simulink model "sm_car"  (R2025b)
settings: Solver=ode23t  StartTime=0.0  StopTime=100  MaxStep=0.4  RelTol=1e-3  AbsTol=1e-3  EnableMultiTasking=on
PreLoadFcn:
  | % Due to usability issue in Repeating Sequence block
  | warning('off','Simulink:Masking:Invalid');
  | 
  | % Eliminate unnecessary warnings in inactive variants
  | % Warnings generated only if you click through inactive variant
  | warning('off','MATLAB:nonExistentField');
  | warning('off','Simulink:Parameters:BlkParamUndefined');
PostLoadFcn:
  | set_param([bdroot '/Vehicle'],'popup_trailer','Off')
  | warning('off','sm:sli:setup:compile:LocalSolverNotSupported')
  | %sm_car_config_maneuver(bdroot,'WOT Braking');
  | sm_car_config_vehicle(bdroot,'false');
  | sm_car_config_logging(bdroot);
InitFcn:
  | sm_car_config_camera;
  | Vehicle = sm_car_vehcfg_checkConfig(Vehicle);
  | sm_car_check_tire_model(bdroot);
StartFcn:
  | tic;
StopFcn:
  | Elapsed_Sim_Time = toc;
  | % disp(['Elapsed Sim Time = ' num2str(Elapsed_Sim_Time)]);
undefined symbols (not defined in the file): Axle1D, AxleIn, Camera, Control, Driver, Init, Maneuver, Pedal, Scene, ShaftL1, ShaftL2, ShaftR1, ShaftR2, Visual, X, xy_data_car_side, Y, Z
libraries: sm_lib x255, fl_lib x191, nesl_utility x149, simulink x23, sdl_lib x14, simulink_extras x8, SimscapeFluids_lib x7, Scene_Utilities x6, Tire_1x2x x4, ee_lib x3, Linkage x2, fuzblock x1
(part 3 of 19)

== system sm_car/Camera Frames/Transform FixO RR ==
  Transform Camera Frame : sm_lib/Frames and Transforms/Rigid Transform  RotationMethod=RotationSequence  FollAlignAxisA=+X  BaseAlignAxisA=+Y  FollAlignAxisB=+Y  BaseAlignAxisB=+Z  RotationStandardAxis=+Z  RotationAngle=0.0  RotationAngleUnits=deg  RotationArbitraryAxis=[0 0 1]  RotationSequenceAxes=FollowerAxes  RotationSequence=ZYX  RotationSequenceAngles=CF.a.Value(3:-1:1)  RotationSequenceAnglesUnits=deg  RotationMatrix=[1 0 0; 0 1 0; 0 0 1]  Quaternion=[1 0 0 0]  TranslationMethod=Cartesian  TranslationCartesianOffset=CF.s.Value  TranslationCartesianOffsetUnits=m  TranslationStandardAxis=+Z  TranslationStandardOffset=0  TranslationStandardOffsetUnits=m  TranslationROffset=0  TranslationROffsetUnits=m  TranslationThetaOffset=0  TranslationThetaOffsetUnits=deg  TranslationZOffset=0  TranslationZOffsetUnits=m
  B : PMIOPort  Side=Left
  F : PMIOPort  Port=2  Side=Right
  connections:
  Transform Camera Frame/RConn1 -- F/RConn1
  Transform Camera Frame/LConn1 -- B/RConn1

== system sm_car/Camera Frames/Transform FixO Rear ==
  Transform Camera Frame : sm_lib/Frames and Transforms/Rigid Transform  RotationMethod=RotationSequence  FollAlignAxisA=+X  BaseAlignAxisA=+Y  FollAlignAxisB=+Y  BaseAlignAxisB=+Z  RotationStandardAxis=+Z  RotationAngle=0.0  RotationAngleUnits=deg  RotationArbitraryAxis=[0 0 1]  RotationSequenceAxes=FollowerAxes  RotationSequence=ZYX  RotationSequenceAngles=CF.a.Value(3:-1:1)  RotationSequenceAnglesUnits=deg  RotationMatrix=[1 0 0; 0 1 0; 0 0 1]  Quaternion=[1 0 0 0]  TranslationMethod=Cartesian  TranslationCartesianOffset=CF.s.Value  TranslationCartesianOffsetUnits=m  TranslationStandardAxis=+Z  TranslationStandardOffset=0  TranslationStandardOffsetUnits=m  TranslationROffset=0  TranslationROffsetUnits=m  TranslationThetaOffset=0  TranslationThetaOffsetUnits=deg  TranslationZOffset=0  TranslationZOffsetUnits=m
  B : PMIOPort  Side=Left
  F : PMIOPort  Port=2  Side=Right
  connections:
  Transform Camera Frame/RConn1 -- F/RConn1
  Transform Camera Frame/LConn1 -- B/RConn1

== system sm_car/Camera Frames/Transform FixO Right ==
  Transform Camera Frame : sm_lib/Frames and Transforms/Rigid Transform  RotationMethod=RotationSequence  FollAlignAxisA=+X  BaseAlignAxisA=+Y  FollAlignAxisB=+Y  BaseAlignAxisB=+Z  RotationStandardAxis=+Z  RotationAngle=0.0  RotationAngleUnits=deg  RotationArbitraryAxis=[0 0 1]  RotationSequenceAxes=FollowerAxes  RotationSequence=ZYX  RotationSequenceAngles=CF.a.Value(3:-1:1)  RotationSequenceAnglesUnits=deg  RotationMatrix=[1 0 0; 0 1 0; 0 0 1]  Quaternion=[1 0 0 0]  TranslationMethod=Cartesian  TranslationCartesianOffset=CF.s.Value  TranslationCartesianOffsetUnits=m  TranslationStandardAxis=+Z  TranslationStandardOffset=0  TranslationStandardOffsetUnits=m  TranslationROffset=0  TranslationROffsetUnits=m  TranslationThetaOffset=0  TranslationThetaOffsetUnits=deg  TranslationZOffset=0  TranslationZOffsetUnits=m
  B : PMIOPort  Side=Left
  F : PMIOPort  Port=2  Side=Right
  connections:
  Transform Camera Frame/RConn1 -- F/RConn1
  Transform Camera Frame/LConn1 -- B/RConn1

== system sm_car/Camera Frames/Transform FixO Top ==
  Transform Camera Frame : sm_lib/Frames and Transforms/Rigid Transform  RotationMethod=RotationSequence  FollAlignAxisA=+X  BaseAlignAxisA=+Y  FollAlignAxisB=+Y  BaseAlignAxisB=+Z  RotationStandardAxis=+Z  RotationAngle=0.0  RotationAngleUnits=deg  RotationArbitraryAxis=[0 0 1]  RotationSequenceAxes=FollowerAxes  RotationSequence=ZYX  RotationSequenceAngles=CF.a.Value(3:-1:1)  RotationSequenceAnglesUnits=deg  RotationMatrix=[1 0 0; 0 1 0; 0 0 1]  Quaternion=[1 0 0 0]  TranslationMethod=Cartesian  TranslationCartesianOffset=CF.s.Value  TranslationCartesianOffsetUnits=m  TranslationStandardAxis=+Z  TranslationStandardOffset=0  TranslationStandardOffsetUnits=m  TranslationROffset=0  TranslationROffsetUnits=m  TranslationThetaOffset=0  TranslationThetaOffsetUnits=deg  TranslationZOffset=0  TranslationZOffsetUnits=m
  B : PMIOPort  Side=Left
  F : PMIOPort  Port=2  Side=Right
  connections:
  Transform Camera Frame/RConn1 -- F/RConn1
  Transform Camera Frame/LConn1 -- B/RConn1

== system sm_car/Camera Frames/Transform Front ==
  Transform Camera Frame : sm_lib/Frames and Transforms/Rigid Transform  RotationMethod=RotationSequence  FollAlignAxisA=+X  BaseAlignAxisA=+Y  FollAlignAxisB=+Y  BaseAlignAxisB=+Z  RotationStandardAxis=+Z  RotationAngle=0.0  RotationAngleUnits=deg  RotationArbitraryAxis=[0 0 1]  RotationSequenceAxes=FollowerAxes  RotationSequence=ZYX  RotationSequenceAngles=CF.a.Value(3:-1:1)  RotationSequenceAnglesUnits=deg  RotationMatrix=[1 0 0; 0 1 0; 0 0 1]  Quaternion=[1 0 0 0]  TranslationMethod=Cartesian  TranslationCartesianOffset=CF.s.Value  TranslationCartesianOffsetUnits=m  TranslationStandardAxis=+Z  TranslationStandardOffset=0  TranslationStandardOffsetUnits=m  TranslationROffset=0  TranslationROffsetUnits=m  TranslationThetaOffset=0  TranslationThetaOffsetUnits=deg  TranslationZOffset=0  TranslationZOffsetUnits=m
  B : PMIOPort  Side=Left
  F : PMIOPort  Port=2  Side=Right
  connections:
  Transform Camera Frame/RConn1 -- F/RConn1
  Transform Camera Frame/LConn1 -- B/RConn1

== system sm_car/Camera Frames/Transform Left ==
  Transform Camera Frame : sm_lib/Frames and Transforms/Rigid Transform  RotationMethod=RotationSequence  FollAlignAxisA=+X  BaseAlignAxisA=+Y  FollAlignAxisB=+Y  BaseAlignAxisB=+Z  RotationStandardAxis=+Z  RotationAngle=0.0  RotationAngleUnits=deg  RotationArbitraryAxis=[0 0 1]  RotationSequenceAxes=FollowerAxes  RotationSequence=ZYX  RotationSequenceAngles=CF.a.Value(3:-1:1)  RotationSequenceAnglesUnits=deg  RotationMatrix=[1 0 0; 0 1 0; 0 0 1]  Quaternion=[1 0 0 0]  TranslationMethod=Cartesian  TranslationCartesianOffset=CF.s.Value  TranslationCartesianOffsetUnits=m  TranslationStandardAxis=+Z  TranslationStandardOffset=0  TranslationStandardOffsetUnits=m  TranslationROffset=0  TranslationROffsetUnits=m  TranslationThetaOffset=0  TranslationThetaOffsetUnits=deg  TranslationZOffset=0  TranslationZOffsetUnits=m
  B : PMIOPort  Side=Left
  F : PMIOPort  Port=2  Side=Right
  connections:
  Transform Camera Frame/RConn1 -- F/RConn1
  Transform Camera Frame/LConn1 -- B/RConn1

== system sm_car/Camera Frames/Transform RL ==
  Transform Camera Frame : sm_lib/Frames and Transforms/Rigid Transform  RotationMethod=RotationSequence  FollAlignAxisA=+X  BaseAlignAxisA=+Y  FollAlignAxisB=+Y  BaseAlignAxisB=+Z  RotationStandardAxis=+Z  RotationAngle=0.0  RotationAngleUnits=deg  RotationArbitraryAxis=[0 0 1]  RotationSequenceAxes=FollowerAxes  RotationSequence=ZYX  RotationSequenceAngles=CF.a.Value(3:-1:1)  RotationSequenceAnglesUnits=deg  RotationMatrix=[1 0 0; 0 1 0; 0 0 1]  Quaternion=[1 0 0 0]  TranslationMethod=Cartesian  TranslationCartesianOffset=CF.s.Value  TranslationCartesianOffsetUnits=m  TranslationStandardAxis=+Z  TranslationStandardOffset=0  TranslationStandardOffsetUnits=m  TranslationROffset=0  TranslationROffsetUnits=m  TranslationThetaOffset=0  TranslationThetaOffsetUnits=deg  TranslationZOffset=0  TranslationZOffsetUnits=m
  B : PMIOPort  Side=Left
  F : PMIOPort  Port=2  Side=Right
  connections:
  Transform Camera Frame/RConn1 -- F/RConn1
  Transform Camera Frame/LConn1 -- B/RConn1

== system sm_car/Camera Frames/Transform RR ==
  Transform Camera Frame : sm_lib/Frames and Transforms/Rigid Transform  RotationMethod=RotationSequence  FollAlignAxisA=+X  BaseAlignAxisA=+Y  FollAlignAxisB=+Y  BaseAlignAxisB=+Z  RotationStandardAxis=+Z  RotationAngle=0.0  RotationAngleUnits=deg  RotationArbitraryAxis=[0 0 1]  RotationSequenceAxes=FollowerAxes  RotationSequence=ZYX  RotationSequenceAngles=CF.a.Value(3:-1:1)  RotationSequenceAnglesUnits=deg  RotationMatrix=[1 0 0; 0 1 0; 0 0 1]  Quaternion=[1 0 0 0]  TranslationMethod=Cartesian  TranslationCartesianOffset=CF.s.Value  TranslationCartesianOffsetUnits=m  TranslationStandardAxis=+Z  TranslationStandardOffset=0  TranslationStandardOffsetUnits=m  TranslationROffset=0  TranslationROffsetUnits=m  TranslationThetaOffset=0  TranslationThetaOffsetUnits=deg  TranslationZOffset=0  TranslationZOffsetUnits=m
  B : PMIOPort  Side=Left
  F : PMIOPort  Port=2  Side=Right
  connections:
  Transform Camera Frame/RConn1 -- F/RConn1
  Transform Camera Frame/LConn1 -- B/RConn1

== system sm_car/Camera Frames/Transform Rear ==
  Transform Camera Frame : sm_lib/Frames and Transforms/Rigid Transform  RotationMethod=RotationSequence  FollAlignAxisA=+X  BaseAlignAxisA=+Y  FollAlignAxisB=+Y  BaseAlignAxisB=+Z  RotationStandardAxis=+Z  RotationAngle=0.0  RotationAngleUnits=deg  RotationArbitraryAxis=[0 0 1]  RotationSequenceAxes=FollowerAxes  RotationSequence=ZYX  RotationSequenceAngles=CF.a.Value(3:-1:1)  RotationSequenceAnglesUnits=deg  RotationMatrix=[1 0 0; 0 1 0; 0 0 1]  Quaternion=[1 0 0 0]  TranslationMethod=Cartesian  TranslationCartesianOffset=CF.s.Value  TranslationCartesianOffsetUnits=m  TranslationStandardAxis=+Z  TranslationStandardOffset=0  TranslationStandardOffsetUnits=m  TranslationROffset=0  TranslationROffsetUnits=m  TranslationThetaOffset=0  TranslationThetaOffsetUnits=deg  TranslationZOffset=0  TranslationZOffsetUnits=m
  B : PMIOPort  Side=Left
  F : PMIOPort  Port=2  Side=Right
  connections:
  Transform Camera Frame/RConn1 -- F/RConn1
  Transform Camera Frame/LConn1 -- B/RConn1

== system sm_car/Camera Frames/Transform Right ==
  Transform Camera Frame : sm_lib/Frames and Transforms/Rigid Transform  RotationMethod=RotationSequence  FollAlignAxisA=+X  BaseAlignAxisA=+Y  FollAlignAxisB=+Y  BaseAlignAxisB=+Z  RotationStandardAxis=+Z  RotationAngle=0.0  RotationAngleUnits=deg  RotationArbitraryAxis=[0 0 1]  RotationSequenceAxes=FollowerAxes  RotationSequence=ZYX  RotationSequenceAngles=CF.a.Value(3:-1:1)  RotationSequenceAnglesUnits=deg  RotationMatrix=[1 0 0; 0 1 0; 0 0 1]  Quaternion=[1 0 0 0]  TranslationMethod=Cartesian  TranslationCartesianOffset=CF.s.Value  TranslationCartesianOffsetUnits=m  TranslationStandardAxis=+Z  TranslationStandardOffset=0  TranslationStandardOffsetUnits=m  TranslationROffset=0  TranslationROffsetUnits=m  TranslationThetaOffset=0  TranslationThetaOffsetUnits=deg  TranslationZOffset=0  TranslationZOffsetUnits=m
  B : PMIOPort  Side=Left
  F : PMIOPort  Port=2  Side=Right
  connections:
  Transform Camera Frame/RConn1 -- F/RConn1
  Transform Camera Frame/LConn1 -- B/RConn1

== system sm_car/Camera Frames/Transform SuspF ==
  Transform Camera Frame : sm_lib/Frames and Transforms/Rigid Transform  RotationMethod=RotationSequence  FollAlignAxisA=+X  BaseAlignAxisA=+Y  FollAlignAxisB=+Y  BaseAlignAxisB=+Z  RotationStandardAxis=+Z  RotationAngle=0.0  RotationAngleUnits=deg  RotationArbitraryAxis=[0 0 1]  RotationSequenceAxes=FollowerAxes  RotationSequence=ZYX  RotationSequenceAngles=CF.a.Value(3:-1:1)  RotationSequenceAnglesUnits=deg  RotationMatrix=[1 0 0; 0 1 0; 0 0 1]  Quaternion=[1 0 0 0]  TranslationMethod=Cartesian  TranslationCartesianOffset=CF.s.Value  TranslationCartesianOffsetUnits=m  TranslationStandardAxis=+Z  TranslationStandardOffset=0  TranslationStandardOffsetUnits=m  TranslationROffset=0  TranslationROffsetUnits=m  TranslationThetaOffset=0  TranslationThetaOffsetUnits=deg  TranslationZOffset=0  TranslationZOffsetUnits=m
  B : PMIOPort  Side=Left
  F : PMIOPort  Port=2  Side=Right
  connections:
  Transform Camera Frame/RConn1 -- F/RConn1
  Transform Camera Frame/LConn1 -- B/RConn1

== system sm_car/Camera Frames/Transform SuspR ==
  Transform Camera Frame : sm_lib/Frames and Transforms/Rigid Transform  RotationMethod=RotationSequence  FollAlignAxisA=+X  BaseAlignAxisA=+Y  FollAlignAxisB=+Y  BaseAlignAxisB=+Z  RotationStandardAxis=+Z  RotationAngle=0.0  RotationAngleUnits=deg  RotationArbitraryAxis=[0 0 1]  RotationSequenceAxes=FollowerAxes  RotationSequence=ZYX  RotationSequenceAngles=CF.a.Value(3:-1:1)  RotationSequenceAnglesUnits=deg  RotationMatrix=[1 0 0; 0 1 0; 0 0 1]  Quaternion=[1 0 0 0]  TranslationMethod=Cartesian  TranslationCartesianOffset=CF.s.Value  TranslationCartesianOffsetUnits=m  TranslationStandardAxis=+Z  TranslationStandardOffset=0  TranslationStandardOffsetUnits=m  TranslationROffset=0  TranslationROffsetUnits=m  TranslationThetaOffset=0  TranslationThetaOffsetUnits=deg  TranslationZOffset=0  TranslationZOffsetUnits=m
  B : PMIOPort  Side=Left
  F : PMIOPort  Port=2  Side=Right
  connections:
  Transform Camera Frame/RConn1 -- F/RConn1
  Transform Camera Frame/LConn1 -- B/RConn1

== system sm_car/Camera Frames/Transform Top ==
  Transform Camera Frame : sm_lib/Frames and Transforms/Rigid Transform  RotationMethod=RotationSequence  FollAlignAxisA=+X  BaseAlignAxisA=+Y  FollAlignAxisB=+Y  BaseAlignAxisB=+Z  RotationStandardAxis=+Z  RotationAngle=0.0  RotationAngleUnits=deg  RotationArbitraryAxis=[0 0 1]  RotationSequenceAxes=FollowerAxes  RotationSequence=ZYX  RotationSequenceAngles=CF.a.Value(3:-1:1)  RotationSequenceAnglesUnits=deg  RotationMatrix=[1 0 0; 0 1 0; 0 0 1]  Quaternion=[1 0 0 0]  TranslationMethod=Cartesian  TranslationCartesianOffset=CF.s.Value  TranslationCartesianOffsetUnits=m  TranslationStandardAxis=+Z  TranslationStandardOffset=0  TranslationStandardOffsetUnits=m  TranslationROffset=0  TranslationROffsetUnits=m  TranslationThetaOffset=0  TranslationThetaOffsetUnits=deg  TranslationZOffset=0  TranslationZOffsetUnits=m
  B : PMIOPort  Side=Left
  F : PMIOPort  Port=2  Side=Right
  connections:
  Transform Camera Frame/RConn1 -- F/RConn1
  Transform Camera Frame/LConn1 -- B/RConn1

== system sm_car/Camera Frames/Transform View Seat FL ==
  Transform Camera Frame : sm_lib/Frames and Transforms/Rigid Transform  RotationMethod=RotationSequence  FollAlignAxisA=+X  BaseAlignAxisA=+Y  FollAlignAxisB=+Y  BaseAlignAxisB=+Z  RotationStandardAxis=+Z  RotationAngle=0.0  RotationAngleUnits=deg  RotationArbitraryAxis=[0 0 1]  RotationSequenceAxes=FollowerAxes  RotationSequence=ZYX  RotationSequenceAngles=CF.a.Value(3:-1:1)  RotationSequenceAnglesUnits=deg  RotationMatrix=[1 0 0; 0 1 0; 0 0 1]  Quaternion=[1 0 0 0]  TranslationMethod=Cartesian  TranslationCartesianOffset=CF.s.Value  TranslationCartesianOffsetUnits=m  TranslationStandardAxis=+Z  TranslationStandardOffset=0  TranslationStandardOffsetUnits=m  TranslationROffset=0  TranslationROffsetUnits=m  TranslationThetaOffset=0  TranslationThetaOffsetUnits=deg  TranslationZOffset=0  TranslationZOffsetUnits=m
  B : PMIOPort  Side=Left
  F : PMIOPort  Port=2  Side=Right
  connections:
  Transform Camera Frame/RConn1 -- F/RConn1
  Transform Camera Frame/LConn1 -- B/RConn1

== system sm_car/Camera Frames/Transform View Seat FR ==
  Transform Camera Frame : sm_lib/Frames and Transforms/Rigid Transform  RotationMethod=RotationSequence  FollAlignAxisA=+X  BaseAlignAxisA=+Y  FollAlignAxisB=+Y  BaseAlignAxisB=+Z  RotationStandardAxis=+Z  RotationAngle=0.0  RotationAngleUnits=deg  RotationArbitraryAxis=[0 0 1]  RotationSequenceAxes=FollowerAxes  RotationSequence=ZYX  RotationSequenceAngles=CF.a.Value(3:-1:1)  RotationSequenceAnglesUnits=deg  RotationMatrix=[1 0 0; 0 1 0; 0 0 1]  Quaternion=[1 0 0 0]  TranslationMethod=Cartesian  TranslationCartesianOffset=CF.s.Value  TranslationCartesianOffsetUnits=m  TranslationStandardAxis=+Z  TranslationStandardOffset=0  TranslationStandardOffsetUnits=m  TranslationROffset=0  TranslationROffsetUnits=m  TranslationThetaOffset=0  TranslationThetaOffsetUnits=deg  TranslationZOffset=0  TranslationZOffsetUnits=m
  B : PMIOPort  Side=Left
  F : PMIOPort  Port=2  Side=Right
  connections:
  Transform Camera Frame/RConn1 -- F/RConn1
  Transform Camera Frame/LConn1 -- B/RConn1

== system sm_car/Camera Frames/Transform View Susp FL ==
  Transform Camera Frame : sm_lib/Frames and Transforms/Rigid Transform  RotationMethod=RotationSequence  FollAlignAxisA=+X  BaseAlignAxisA=+Y  FollAlignAxisB=+Y  BaseAlignAxisB=+Z  RotationStandardAxis=+Z  RotationAngle=0.0  RotationAngleUnits=deg  RotationArbitraryAxis=[0 0 1]  RotationSequenceAxes=FollowerAxes  RotationSequence=ZYX  RotationSequenceAngles=CF.a.Value(3:-1:1)  RotationSequenceAnglesUnits=deg  RotationMatrix=[1 0 0; 0 1 0; 0 0 1]  Quaternion=[1 0 0 0]  TranslationMethod=Cartesian  TranslationCartesianOffset=CF.s.Value  TranslationCartesianOffsetUnits=m  TranslationStandardAxis=+Z  TranslationStandardOffset=0  TranslationStandardOffsetUnits=m  TranslationROffset=0  TranslationROffsetUnits=m  TranslationThetaOffset=0  TranslationThetaOffsetUnits=deg  TranslationZOffset=0  TranslationZOffsetUnits=m
  B : PMIOPort  Side=Left
  F : PMIOPort  Port=2  Side=Right
  connections:
  Transform Camera Frame/RConn1 -- F/RConn1
  Transform Camera Frame/LConn1 -- B/RConn1

== system sm_car/Camera Frames/Transform View Susp FR ==
  Transform Camera Frame : sm_lib/Frames and Transforms/Rigid Transform  RotationMethod=RotationSequence  FollAlignAxisA=+X  BaseAlignAxisA=+Y  FollAlignAxisB=+Y  BaseAlignAxisB=+Z  RotationStandardAxis=+Z  RotationAngle=0.0  RotationAngleUnits=deg  RotationArbitraryAxis=[0 0 1]  RotationSequenceAxes=FollowerAxes  RotationSequence=ZYX  RotationSequenceAngles=CF.a.Value(3:-1:1)  RotationSequenceAnglesUnits=deg  RotationMatrix=[1 0 0; 0 1 0; 0 0 1]  Quaternion=[1 0 0 0]  TranslationMethod=Cartesian  TranslationCartesianOffset=CF.s.Value  TranslationCartesianOffsetUnits=m  TranslationStandardAxis=+Z  TranslationStandardOffset=0  TranslationStandardOffsetUnits=m  TranslationROffset=0  TranslationROffsetUnits=m  TranslationThetaOffset=0  TranslationThetaOffsetUnits=deg  TranslationZOffset=0  TranslationZOffsetUnits=m
  B : PMIOPort  Side=Left
  F : PMIOPort  Port=2  Side=Right
  connections:
  Transform Camera Frame/RConn1 -- F/RConn1
  Transform Camera Frame/LConn1 -- B/RConn1

== system sm_car/Camera Frames/Transform View Susp RL ==
  Transform Camera Frame : sm_lib/Frames and Transforms/Rigid Transform  RotationMethod=RotationSequence  FollAlignAxisA=+X  BaseAlignAxisA=+Y  FollAlignAxisB=+Y  BaseAlignAxisB=+Z  RotationStandardAxis=+Z  RotationAngle=0.0  RotationAngleUnits=deg  RotationArbitraryAxis=[0 0 1]  RotationSequenceAxes=FollowerAxes  RotationSequence=ZYX  RotationSequenceAngles=CF.a.Value(3:-1:1)  RotationSequenceAnglesUnits=deg  RotationMatrix=[1 0 0; 0 1 0; 0 0 1]  Quaternion=[1 0 0 0]  TranslationMethod=Cartesian  TranslationCartesianOffset=CF.s.Value  TranslationCartesianOffsetUnits=m  TranslationStandardAxis=+Z  TranslationStandardOffset=0  TranslationStandardOffsetUnits=m  TranslationROffset=0  TranslationROffsetUnits=m  TranslationThetaOffset=0  TranslationThetaOffsetUnits=deg  TranslationZOffset=0  TranslationZOffsetUnits=m
  B : PMIOPort  Side=Left
  F : PMIOPort  Port=2  Side=Right
  connections:
  Transform Camera Frame/RConn1 -- F/RConn1
  Transform Camera Frame/LConn1 -- B/RConn1

== system sm_car/Camera Frames/Transform View Susp RR ==
  Transform Camera Frame : sm_lib/Frames and Transforms/Rigid Transform  RotationMethod=RotationSequence  FollAlignAxisA=+X  BaseAlignAxisA=+Y  FollAlignAxisB=+Y  BaseAlignAxisB=+Z  RotationStandardAxis=+Z  RotationAngle=0.0  RotationAngleUnits=deg  RotationArbitraryAxis=[0 0 1]  RotationSequenceAxes=FollowerAxes  RotationSequence=ZYX  RotationSequenceAngles=CF.a.Value(3:-1:1)  RotationSequenceAnglesUnits=deg  RotationMatrix=[1 0 0; 0 1 0; 0 0 1]  Quaternion=[1 0 0 0]  TranslationMethod=Cartesian  TranslationCartesianOffset=CF.s.Value  TranslationCartesianOffsetUnits=m  TranslationStandardAxis=+Z  TranslationStandardOffset=0  TranslationStandardOffsetUnits=m  TranslationROffset=0  TranslationROffsetUnits=m  TranslationThetaOffset=0  TranslationThetaOffsetUnits=deg  TranslationZOffset=0  TranslationZOffsetUnits=m
  B : PMIOPort  Side=Left
  F : PMIOPort  Port=2  Side=Right
  connections:
  Transform Camera Frame/RConn1 -- F/RConn1
  Transform Camera Frame/LConn1 -- B/RConn1

== system sm_car/Camera Frames/Transform Wheel FL ==
  Transform Camera Frame : sm_lib/Frames and Transforms/Rigid Transform  RotationMethod=RotationSequence  FollAlignAxisA=+X  BaseAlignAxisA=+Y  FollAlignAxisB=+Y  BaseAlignAxisB=+Z  RotationStandardAxis=+Z  RotationAngle=0.0  RotationAngleUnits=deg  RotationArbitraryAxis=[0 0 1]  RotationSequenceAxes=FollowerAxes  RotationSequence=ZYX  RotationSequenceAngles=CF.a.Value(3:-1:1)  RotationSequenceAnglesUnits=deg  RotationMatrix=[1 0 0; 0 1 0; 0 0 1]  Quaternion=[1 0 0 0]  TranslationMethod=Cartesian  TranslationCartesianOffset=CF.s.Value  TranslationCartesianOffsetUnits=m  TranslationStandardAxis=+Z  TranslationStandardOffset=0  TranslationStandardOffsetUnits=m  TranslationROffset=0  TranslationROffsetUnits=m  TranslationThetaOffset=0  TranslationThetaOffsetUnits=deg  TranslationZOffset=0  TranslationZOffsetUnits=m
  B : PMIOPort  Side=Left
  F : PMIOPort  Port=2  Side=Right
  connections:
  Transform Camera Frame/RConn1 -- F/RConn1
  Transform Camera Frame/LConn1 -- B/RConn1

== system sm_car/Camera Frames/Transform Wheel FR ==
  Transform Camera Frame : sm_lib/Frames and Transforms/Rigid Transform  RotationMethod=RotationSequence  FollAlignAxisA=+X  BaseAlignAxisA=+Y  FollAlignAxisB=+Y  BaseAlignAxisB=+Z  RotationStandardAxis=+Z  RotationAngle=0.0  RotationAngleUnits=deg  RotationArbitraryAxis=[0 0 1]  RotationSequenceAxes=FollowerAxes  RotationSequence=ZYX  RotationSequenceAngles=CF.a.Value(3:-1:1)  RotationSequenceAnglesUnits=deg  RotationMatrix=[1 0 0; 0 1 0; 0 0 1]  Quaternion=[1 0 0 0]  TranslationMethod=Cartesian  TranslationCartesianOffset=CF.s.Value  TranslationCartesianOffsetUnits=m  TranslationStandardAxis=+Z  TranslationStandardOffset=0  TranslationStandardOffsetUnits=m  TranslationROffset=0  TranslationROffsetUnits=m  TranslationThetaOffset=0  TranslationThetaOffsetUnits=deg  TranslationZOffset=0  TranslationZOffsetUnits=m
  B : PMIOPort  Side=Left
  F : PMIOPort  Port=2  Side=Right
  connections:
  Transform Camera Frame/RConn1 -- F/RConn1
  Transform Camera Frame/LConn1 -- B/RConn1

== system sm_car/Camera Frames/Transform Wheel RL ==
  Transform Camera Frame : sm_lib/Frames and Transforms/Rigid Transform  RotationMethod=RotationSequence  FollAlignAxisA=+X  BaseAlignAxisA=+Y  FollAlignAxisB=+Y  BaseAlignAxisB=+Z  RotationStandardAxis=+Z  RotationAngle=0.0  RotationAngleUnits=deg  RotationArbitraryAxis=[0 0 1]  RotationSequenceAxes=FollowerAxes  RotationSequence=ZYX  RotationSequenceAngles=CF.a.Value(3:-1:1)  RotationSequenceAnglesUnits=deg  RotationMatrix=[1 0 0; 0 1 0; 0 0 1]  Quaternion=[1 0 0 0]  TranslationMethod=Cartesian  TranslationCartesianOffset=CF.s.Value  TranslationCartesianOffsetUnits=m  TranslationStandardAxis=+Z  TranslationStandardOffset=0  TranslationStandardOffsetUnits=m  TranslationROffset=0  TranslationROffsetUnits=m  TranslationThetaOffset=0  TranslationThetaOffsetUnits=deg  TranslationZOffset=0  TranslationZOffsetUnits=m
  B : PMIOPort  Side=Left
  F : PMIOPort  Port=2  Side=Right
  connections:
  Transform Camera Frame/RConn1 -- F/RConn1
  Transform Camera Frame/LConn1 -- B/RConn1

== system sm_car/Camera Frames/Transform Wheel RR ==
  Transform Camera Frame : sm_lib/Frames and Transforms/Rigid Transform  RotationMethod=RotationSequence  FollAlignAxisA=+X  BaseAlignAxisA=+Y  FollAlignAxisB=+Y  BaseAlignAxisB=+Z  RotationStandardAxis=+Z  RotationAngle=0.0  RotationAngleUnits=deg  RotationArbitraryAxis=[0 0 1]  RotationSequenceAxes=FollowerAxes  RotationSequence=ZYX  RotationSequenceAngles=CF.a.Value(3:-1:1)  RotationSequenceAnglesUnits=deg  RotationMatrix=[1 0 0; 0 1 0; 0 0 1]  Quaternion=[1 0 0 0]  TranslationMethod=Cartesian  TranslationCartesianOffset=CF.s.Value  TranslationCartesianOffsetUnits=m  TranslationStandardAxis=+Z  TranslationStandardOffset=0  TranslationStandardOffsetUnits=m  TranslationROffset=0  TranslationROffsetUnits=m  TranslationThetaOffset=0  TranslationThetaOffsetUnits=deg  TranslationZOffset=0  TranslationZOffsetUnits=m
  B : PMIOPort  Side=Left
  F : PMIOPort  Port=2  Side=Right
  connections:
  Transform Camera Frame/RConn1 -- F/RConn1
  Transform Camera Frame/LConn1 -- B/RConn1

== system sm_car/Controller/Default ==
  DrvBus : Inport
  VehBus : Inport  Port=2
  Brake Control : Subsystem  Variant=on  VariantControlMode=label  VariantControl=Variant1  LabelModeActiveChoice=Pedal  mask{popup_brake_control=Pedal, abs_tire_radiusF=Vehicle.Chassis.Tire.tire_radius.Value, abs_tire_radiusR=Vehicle.Chassis.Tire.tire_radius.Value}
      mask prompts: popup_brake_control "Control Type"; abs_tire_radiusF "Tire Radius Front (m)"; abs_tire_radiusR "Tire Radius Rear (m)"
      mask init:
      | set_param(gcb,'LabelModeActiveChoice',get_param(gcb,'popup_brake_control'));
      settings: AttributesFormatString=%<ActiveVariant>
      mask TypeOptions popup_brake_control: Pedal | Pressure | ABS
      mask Display: disp(' ');
  Bus Creator1 : BusCreator  Inputs=4
  Bus Creator2 : BusCreator  Inputs=4
  Bus Selector : BusSelector  OutputSignals=Chassis.Body.CG.vx
  Bus Selector1 : BusSelector  OutputSignals=aSteerWheel,rAccelPedal,rBrakePedal
  Driveline Control : Subsystem
  Power Control : Subsystem  mask{trq_max=Control.Default.maxTrqRequest, trq_ratio_front=Control.Default.pcnt_torque_on_f, trq_rate_up=300, trq_rate_down=-5000}
      mask prompts: trq_max "Max Torque Request"; trq_ratio_front "Ratio of Torque on Front Wheels (0-1)"; trq_rate_up "Torque Rate Limit Up (N*m/s)"; trq_rate_down "Torque Rate Limit Down (N*m/s)"
  Spring Damper : Subsystem
  Susp : Subsystem  mask{Steer=Control.Default.Steer}
      mask prompts: Steer "Steer (structure)"
  CtrlBus : Outport  VectorParamsAs1DForOutWhenUnconnected=off
  wires:
  DrvBus/1 -> Bus Selector1/1
  Bus Creator2/1 -> CtrlBus/1  "CtrlBus"
  Bus Selector1/3 -> Brake Control/1("rBrakePedal ")  "<rBrakePedal>"
  Bus Selector1/2 -> Power Control/1(rAccelPedal)  "<rAccelPedal>"
  Spring Damper/2(Spring) -> Bus Creator1/4
  Power Control/1(Power) -> Bus Creator2/2
  Driveline Control/1(Driveline) -> Bus Creator2/3
  Spring Damper/1(Damper) -> Bus Creator1/3
  Bus Creator1/1 -> Bus Creator2/1  "Chassis"
  Brake Control/1(" Brakes") -> Bus Creator2/4
  Susp/1(SuspA1) -> Bus Creator1/1
  VehBus/1 -> Power Control/2(VehBus), Brake Control/2("VehBus "), Bus Selector/1
  Susp/2(SuspA2) -> Bus Creator1/2
  Bus Selector1/1 -> Susp/1(aSteerWheel)  "<aSteerWheel>"
  Bus Selector/1 -> Susp/2(vx)  "<vx>"

== system sm_car/Controller/FeedF_Ctrl ==
  DrvBus : Inport
  VehBus : Inport  Port=2
  Brake Control : Subsystem  Variant=on  VariantControlMode=label  VariantControl=Variant1  LabelModeActiveChoice=Pedal  mask{popup_brake_control=Pedal, abs_tire_radiusF=Vehicle.Chassis.TireA1.tire_radius.Value, abs_tire_radiusR=Vehicle.Chassis.TireA2.tire_radius.Value}
      mask prompts: popup_brake_control "Control Type"; abs_tire_radiusF "Tire Radius Front (m)"; abs_tire_radiusR "Tire Radius Rear (m)"
      mask init:
      | set_param(gcb,'LabelModeActiveChoice',get_param(gcb,'popup_brake_control'));
      settings: AttributesFormatString=%<ActiveVariant>
      mask TypeOptions popup_brake_control: Pedal | Pressure | ABS
      mask Display: disp(' ');
  Bus Creator1 : BusCreator  Inputs=4
  Bus Creator2 : BusCreator  Inputs=4
  Bus Selector : BusSelector  OutputSignals=Chassis.Body.CG.vx
  Bus Selector1 : BusSelector  OutputSignals=aSteerWheel,rAccelPedal,rBrakePedal
  Driveline Control : Subsystem
  Power Control : Subsystem  mask{Control=Control}
      mask prompts: Control "Control Parameters"
  Spring Damper : Subsystem
  Susp : Subsystem  mask{Steer=Control.Steer}
      mask prompts: Steer "Steer (structure)"
  CtrlBus : Outport  VectorParamsAs1DForOutWhenUnconnected=off
  wires:
  Bus Selector/1 -> Susp/2(vx)  "<vx>"
  Bus Selector1/1 -> Susp/1(aSteerWheel), Power Control/3(aSteerWheel)  "<aSteerWheel>"
  Susp/2(SuspA2) -> Bus Creator1/2
  VehBus/1 -> Bus Selector/1, Brake Control/2("VehBus "), Power Control/2(VehBus)
  Susp/1(SuspA1) -> Bus Creator1/1
  Brake Control/1(" Brakes") -> Bus Creator2/4
  Bus Creator1/1 -> Bus Creator2/1  "Chassis"
  Spring Damper/1(Damper) -> Bus Creator1/3
  Driveline Control/1(Driveline) -> Bus Creator2/3
  Power Control/1(Power) -> Bus Creator2/2  "Power"
  Spring Damper/2(Spring) -> Bus Creator1/4
  Bus Selector1/2 -> Power Control/1(rAccelPedal)  "<rAccelPedal>"
  Bus Selector1/3 -> Brake Control/1("rBrakePedal ")  "<rBrakePedal>"
  Bus Creator2/1 -> CtrlBus/1  "CtrlBus"
  DrvBus/1 -> Bus Selector1/1

== system sm_car/Controller/NoIMU ==
  DrvBus : Inport
  VehBus : Inport  Port=2
  Brake Control : Subsystem  Variant=on  VariantControlMode=label  VariantControl=Variant1  LabelModeActiveChoice=Pedal  mask{popup_brake_control=Pedal, abs_tire_radiusF=Vehicle.Chassis.TireA1.tire_radius.Value, abs_tire_radiusR=Vehicle.Chassis.TireA2.tire_radius.Value}
      mask prompts: popup_brake_control "Control Type"; abs_tire_radiusF "Tire Radius Front (m)"; abs_tire_radiusR "Tire Radius Rear (m)"
      mask init:
      | set_param(gcb,'LabelModeActiveChoice',get_param(gcb,'popup_brake_control'));
      settings: AttributesFormatString=%<ActiveVariant>
      mask TypeOptions popup_brake_control: Pedal | Pressure | ABS
      mask Display: disp(' ');
  Bus Creator1 : BusCreator  Inputs=4
  Bus Creator2 : BusCreator  Inputs=4
  Bus Selector : BusSelector  OutputSignals=Chassis.Body.CG.vx
  Bus Selector1 : BusSelector  OutputSignals=aSteerWheel,rAccelPedal,rBrakePedal
  Driveline Control : Subsystem
  Power Control : Subsystem  mask(Control system parameters){Km=Control.NoIMU.CurrentTrqConst, Tmax=Control.NoIMU.Tmax, I0=Control.NoIMU.I0Load, w0=Control.NoIMU.wLoad, fis=Control.NoIMU.FuzzySystem}
      mask prompts: Km "Motor current-torque const"; Tmax "Max Torque"; I0 "No Load Current"; w0 "No Load RPM"; fis "Fuzzy System"
  Spring Damper : Subsystem
  Susp : Subsystem  mask{Steer=Control.Default.Steer}
      mask prompts: Steer "Steer (structure)"
  CtrlBus : Outport  VectorParamsAs1DForOutWhenUnconnected=off
  wires:
  Bus Selector/1 -> Susp/2(vx)  "<vx>"
  Bus Selector1/1 -> Susp/1(aSteerWheel)  "<aSteerWheel>"
  Susp/2(SuspA2) -> Bus Creator1/2
  VehBus/1 -> Bus Selector/1, Brake Control/2("VehBus "), Power Control/2(VehBus)
  Susp/1(SuspA1) -> Bus Creator1/1
  Brake Control/1(" Brakes") -> Bus Creator2/4
  Bus Creator1/1 -> Bus Creator2/1  "Chassis"
  Spring Damper/1(Damper) -> Bus Creator1/3
  Driveline Control/1(Driveline) -> Bus Creator2/3
  Power Control/1(Power) -> Bus Creator2/2
  Spring Damper/2(Spring) -> Bus Creator1/4
  Bus Selector1/2 -> Power Control/1(rAccelPedal)  "<rAccelPedal>"
  Bus Selector1/3 -> Brake Control/1("rBrakePedal ")  "<rBrakePedal>"
  Bus Creator2/1 -> CtrlBus/1  "CtrlBus"
  DrvBus/1 -> Bus Selector1/1

== system sm_car/Controller/Slip_Ctrl ==
  DrvBus : Inport
  VehBus : Inport  Port=2
  Brake Control : Subsystem  Variant=on  VariantControlMode=label  VariantControl=Variant1  LabelModeActiveChoice=Pedal  mask{popup_brake_control=Pedal, abs_tire_radiusF=Vehicle.Chassis.Tire.tire_radius.Value}
      mask prompts: popup_brake_control "Control Type"; abs_tire_radiusF "Tire Radius (m)"
      mask init:
      | set_param(gcb,'LabelModeActiveChoice',get_param(gcb,'popup_brake_control'));
      settings: AttributesFormatString=%<ActiveVariant>
      mask TypeOptions popup_brake_control: Pedal | Pressure | ABS
      mask Display: disp(' ');
  Bus Creator1 : BusCreator  Inputs=4
  Bus Creator2 : BusCreator  Inputs=4
  Bus Selector : BusSelector  OutputSignals=Chassis.Body.CG.vx
  Bus Selector1 : BusSelector  OutputSignals=aSteerWheel,rAccelPedal,rBrakePedal
  Driveline Control : Subsystem
  Power Control : Subsystem  mask{Control=Control}
      mask prompts: Control "Control Parameters"
  Spring Damper : Subsystem
  Susp : Subsystem  mask{Steer=Control.Steer}
      mask prompts: Steer "Steer (structure)"
  CtrlBus : Outport  VectorParamsAs1DForOutWhenUnconnected=off
  wires:
  Bus Selector/1 -> Susp/2(vx)  "<vx>"
  Bus Selector1/1 -> Susp/1(aSteerWheel)  "<aSteerWheel>"
  Susp/2(SuspA2) -> Bus Creator1/2
  VehBus/1 -> Bus Selector/1, Brake Control/2("VehBus "), Power Control/2(VehBus)
  Susp/1(SuspA1) -> Bus Creator1/1
  Brake Control/1(" Brakes") -> Bus Creator2/4
  Bus Creator1/1 -> Bus Creator2/1  "Chassis"
  Spring Damper/1(Damper) -> Bus Creator1/3
  Driveline Control/1(Driveline) -> Bus Creator2/3
  Power Control/1(Power) -> Bus Creator2/2  "Power"
  Spring Damper/2(Spring) -> Bus Creator1/4
  Bus Selector1/2 -> Power Control/1(rAccelPedal)  "<rAccelPedal>"
  Bus Selector1/3 -> Brake Control/1("rBrakePedal ")  "<rBrakePedal>"
  Bus Creator2/1 -> CtrlBus/1  "CtrlBus"
  DrvBus/1 -> Bus Selector1/1

== system sm_car/Controller/TrqVec 4Motor ==
  DrvBus : Inport
  VehBus : Inport  Port=2
  Brake Control : Subsystem  Variant=on  VariantControlMode=label  VariantControl=Variant1  LabelModeActiveChoice=Pedal  mask{popup_brake_control=Pedal, abs_tire_radiusF=Vehicle.Chassis.TireA1.tire_radius.Value, abs_tire_radiusR=Vehicle.Chassis.TireA2.tire_radius.Value}
      mask prompts: popup_brake_control "Control Type"; abs_tire_radiusF "Tire Radius Front (m)"; abs_tire_radiusR "Tire Radius Rear (m)"
      mask init:
      | set_param(gcb,'LabelModeActiveChoice',get_param(gcb,'popup_brake_control'));
      settings: AttributesFormatString=%<ActiveVariant>
      mask TypeOptions popup_brake_control: Pedal | Pressure | ABS
      mask Display: disp(' ');
  Bus Creator1 : BusCreator  Inputs=4
  Bus Creator2 : BusCreator  Inputs=4
  Bus Selector : BusSelector  OutputSignals=aSteerWheel
  Bus Selector1 : BusSelector  OutputSignals=rBrakePedal
  Bus Selector2 : BusSelector  OutputSignals=Chassis.Body.CG.vx
  Driveline Control : Subsystem
  Power_TqVec : Subsystem  mask{Control=Control.TrqVec}
      mask prompts: Control "Control Parameters"
  Spring Damper : Subsystem
  Susp : Subsystem  mask{Steer=Control.Default.Steer}
      mask prompts: Steer "Steer (structure)"
  CtrlBus : Outport  VectorParamsAs1DForOutWhenUnconnected=off
  wires:
  Bus Selector2/1 -> Susp/2(vx)  "<vx>"
  Bus Selector/1 -> Susp/1(aSteerWheel)  "<aSteerWheel>"
  DrvBus/1 -> Bus Selector/1, Power_TqVec/1(DrvBus), Bus Selector1/1
  Bus Creator2/1 -> CtrlBus/1  "CtrlBus"
  Bus Selector1/1 -> Brake Control/1("rBrakePedal ")  "<rBrakePedal>"
  Spring Damper/2(Spring) -> Bus Creator1/4
  Power_TqVec/1(Power) -> Bus Creator2/2
  Driveline Control/1(Driveline) -> Bus Creator2/3
  Spring Damper/1(Damper) -> Bus Creator1/3
  Bus Creator1/1 -> Bus Creator2/1  "Chassis"
  Brake Control/1(" Brakes") -> Bus Creator2/4
  Susp/1(SuspA1) -> Bus Creator1/1
  VehBus/1 -> Brake Control/2("VehBus "), Power_TqVec/2(VehBus), Bus Selector2/1
  Susp/2(SuspA2) -> Bus Creator1/2

== system sm_car/Controller/TrqVec_FLC ==
  DrvBus : Inport
  VehBus : Inport  Port=2
  Brake Control : Subsystem  Variant=on  VariantControlMode=label  VariantControl=Variant1  LabelModeActiveChoice=Pedal  mask{popup_brake_control=Pedal, abs_tire_radiusF=Vehicle.Chassis.TireA1.tire_radius.Value, abs_tire_radiusR=Vehicle.Chassis.TireA2.tire_radius.Value}
      mask prompts: popup_brake_control "Control Type"; abs_tire_radiusF "Tire Radius Front (m)"; abs_tire_radiusR "Tire Radius Rear (m)"
      mask init:
      | set_param(gcb,'LabelModeActiveChoice',get_param(gcb,'popup_brake_control'));
      settings: AttributesFormatString=%<ActiveVariant>
      mask TypeOptions popup_brake_control: Pedal | Pressure | ABS
      mask Display: disp(' ');
  Bus Creator1 : BusCreator  Inputs=4
  Bus Creator2 : BusCreator  Inputs=4
  Bus Selector : BusSelector  OutputSignals=Chassis.Body.CG.vx
  Bus Selector1 : BusSelector  OutputSignals=aSteerWheel,rAccelPedal,rBrakePedal
  Driveline Control : Subsystem
  Power Control : Subsystem  mask{Control=Control}
      mask prompts: Control "Control Parameters"
  Spring Damper : Subsystem
  Susp : Subsystem  mask{Steer=Control.Steer}
      mask prompts: Steer "Steer (structure)"
  CtrlBus : Outport  VectorParamsAs1DForOutWhenUnconnected=off
  wires:
  DrvBus/1 -> Bus Selector1/1
  Bus Creator2/1 -> CtrlBus/1  "CtrlBus"
  Bus Selector1/3 -> Brake Control/1("rBrakePedal ")  "<rBrakePedal>"
  Bus Selector1/2 -> Power Control/1(rAccelPedal)  "<rAccelPedal>"
  Spring Damper/2(Spring) -> Bus Creator1/4
  Power Control/1(Power) -> Bus Creator2/2  "Power"
  Driveline Control/1(Driveline) -> Bus Creator2/3
  Spring Damper/1(Damper) -> Bus Creator1/3
  Bus Creator1/1 -> Bus Creator2/1  "Chassis"
  Brake Control/1(" Brakes") -> Bus Creator2/4
  Susp/1(SuspA1) -> Bus Creator1/1
  VehBus/1 -> Power Control/2(VehBus), Brake Control/2("VehBus "), Bus Selector/1
  Susp/2(SuspA2) -> Bus Creator1/2
  Bus Selector1/1 -> Power Control/3(aSteerWheel), Susp/1(aSteerWheel)  "<aSteerWheel>"
  Bus Selector/1 -> Susp/2(vx)  "<vx>"

== system sm_car/Driver/Closed Loop ==
  VehBus : Inport
  Obs : Inport  Port=2
  Bus Selector : BusSelector  OutputSignals=Chassis.Body.CG.vx
  Bus Selector2 : BusSelector  OutputSignals=dist
  Driver : Subsystem  mask(Driver Behavior){Driver=Driver}
      mask help: Models driver behavior to follow prescribed vehicle trajectory, including path and speed.
  Maneuver : Subsystem  mask(Maneuver Follow Trajectory){Maneuver=Maneuver, Value=Maneuver.vGain.Value, popup_window=Yes}
      mask prompts: Value "vGain"; popup_window "Check only window of trajectory"
      mask help: Determines target pose to follow prescribed trajectory. Prescribed trajectory is vehicle pose (x, y, theta) and speed along the path to be followed. Optional visual of target pose is also provided.
      mask init:
      | if(strcmpi(get_param(gcb,'popup_window'),'yes'))
      |     set_param([gcb '/window only'],'Value','1');
      | else
      |     set_param([gcb '/window only'],'Value','0');
      | end
      mask TypeOptions Value: Target Speed Gain/Value
      mask TypeOptions popup_window: No | Yes
  Override : Subsystem  Variant=on  VariantControlMode=label  VariantControl=Variant1  LabelModeActiveChoice=None  mask(Driver Override){popup_override_type=None}
      mask prompts: popup_override_type "Override Type"
      mask help: Optionally override driver commands based on objects in scene. For example, the state of a traffic light can override driver commands to follow a prescribed speed trajectory.
      mask init:
      | set_param(gcb,'LabelModeActiveChoice',strrep(get_param(gcb,'popup_override_type'),' ','_'));
      settings: AttributesFormatString=%<LabelModeActiveChoice>
      mask TypeOptions popup_override_type: None | Track Mallory Park Obstacle
      mask Display: disp(' ');
  Scopes : Subsystem
  Terminator : Terminator
  Transfer Fcn : TransferFcn  Denominator=[0.1 1]
  DrvBus : Outport  VectorParamsAs1DForOutWhenUnconnected=off
  wires:
  Transfer Fcn/1 -> Override/1("dist ")
  Override/1(" Ovr") -> Maneuver/2(Override)
  Bus Selector2/1 -> Transfer Fcn/1  "<dist>"
  Obs/1 -> Override/2("Obs ")
  Maneuver/3(simres) -> Terminator/1
  Driver/1(DrvBus) -> DrvBus/1, Scopes/4(DrvBus)
  Maneuver/2(CurPose) -> Scopes/3(CurPose), Driver/3(CurPose)
  Bus Selector/1 -> Scopes/1(<vx>), Driver/1(vx)  "<vx>"
  VehBus/1 -> Bus Selector/1, Maneuver/1(VehBus)
  Maneuver/1(Ref) -> Scopes/2(Ref), Bus Selector2/1, Driver/2(Ref)

== system sm_car/Driver/Open Loop ==
  VehBus : Inport
  Obs : Inport  Port=2
  Open Loop : Subsystem  mask{Maneuver=Maneuver}
      mask init:
      | X = [0 0];
      | Y = [0 0];
  Terminator : Terminator
  Terminator1 : Terminator
  DrvBus : Outport  VectorParamsAs1DForOutWhenUnconnected=off
  wires:
  Obs/1 -> Terminator1/1
  VehBus/1 -> Terminator/1
  Open Loop/1(DrvBus) -> DrvBus/1

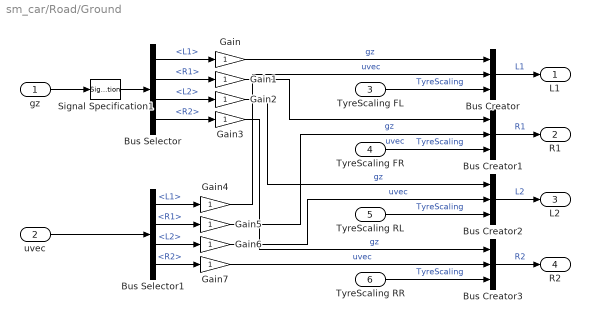
== system sm_car/Road/Ground ==
  gz : Inport
  uvec : Inport  Port=2
  TyreScaling FL : Inport  Port=3
  TyreScaling FR : Inport  Port=4
  TyreScaling RL : Inport  Port=5
  TyreScaling RR : Inport  Port=6
  Bus Creator{,1..3} (4 alike) : BusCreator  Inputs=3
  Bus Selector : BusSelector  OutputSignals=L1,R1,L2,R2
  Bus Selector1 : BusSelector  OutputSignals=L1,R1,L2,R2
  Gain{,1..7} (8 alike) : Gain
  Signal Specification1 : SignalSpecification  Unit=m
  L1 : Outport  VectorParamsAs1DForOutWhenUnconnected=off
  R1 : Outport  Port=2  VectorParamsAs1DForOutWhenUnconnected=off
  L2 : Outport  Port=3  VectorParamsAs1DForOutWhenUnconnected=off
  R2 : Outport  Port=4  VectorParamsAs1DForOutWhenUnconnected=off
  wires:
  Bus Creator/1 -> L1/1  "L1"
  Bus Creator1/1 -> R1/1  "R1"
  Gain1/1 -> Bus Creator1/1  "gz"
  TyreScaling FL/1 -> Bus Creator/3  "TyreScaling"
  Bus Creator3/1 -> R2/1  "R2"
  gz/1 -> Signal Specification1/1
  Gain3/1 -> Bus Creator3/1  "gz"
  Bus Creator2/1 -> L2/1  "L2"
  Signal Specification1/1 -> Bus Selector/1
  Gain2/1 -> Bus Creator2/1  "gz"
  TyreScaling FR/1 -> Bus Creator1/3  "TyreScaling"
  TyreScaling RL/1 -> Bus Creator2/3  "TyreScaling"
  TyreScaling RR/1 -> Bus Creator3/3  "TyreScaling"
  Bus Selector/1 -> Gain/1  "<L1>"
  Gain/1 -> Bus Creator/1  "gz"
  Bus Selector/2 -> Gain1/1  "<R1>"
  Bus Selector/3 -> Gain2/1  "<L2>"
  Bus Selector/4 -> Gain3/1  "<R2>"
  uvec/1 -> Bus Selector1/1
  Bus Selector1/1 -> Gain4/1  "<L1>"
  Bus Selector1/2 -> Gain5/1  "<R1>"
  Bus Selector1/3 -> Gain6/1  "<L2>"
  Bus Selector1/4 -> Gain7/1  "<R2>"
  Gain4/1 -> Bus Creator/2  "uvec"
  Gain5/1 -> Bus Creator1/2  "uvec"
  Gain6/1 -> Bus Creator2/2  "uvec"
  Gain7/1 -> Bus Creator3/2  "uvec"

== system sm_car/Road/Input fWindCar ==
  Bus Creator1 : BusCreator  Inputs=3
  Demux : Demux  Outputs=3
  Step : Step  Time=dWind  After=fWind  SampleTime=0
  Step1 : Step  Time=dWind+tWind  After=fWind  SampleTime=0
  Sum : Sum  Inputs=|+-
  fWind : Outport  VectorParamsAs1DForOutWhenUnconnected=off
  wires:
  Demux/2 -> Bus Creator1/2  "fy"
  Demux/1 -> Bus Creator1/1  "fx"
  Demux/3 -> Bus Creator1/3  "fz"
  Bus Creator1/1 -> fWind/1
  Step/1 -> Sum/1
  Step1/1 -> Sum/2
  Sum/1 -> Demux/1

== system sm_car/Road/Input fWindTrailer ==
  Bus Creator1 : BusCreator  Inputs=3
  Demux : Demux  Outputs=3
  Scope : Scope
      settings: ActiveDisplayYMinimum=-1  ActiveDisplayYMaximum=1
  Step : Step  Time=dWind  After=fWind  SampleTime=0
  Step1 : Step  Time=dWind+tWind  After=fWind  SampleTime=0
  Sum : Sum  Inputs=|+-
  fWind : Outport  VectorParamsAs1DForOutWhenUnconnected=off
  wires:
  Bus Creator1/1 -> fWind/1
  Demux/3 -> Bus Creator1/3  "fz"
  Demux/1 -> Bus Creator1/1  "fx"
  Demux/2 -> Bus Creator1/2  "fy"
  Sum/1 -> Scope/1, Demux/1  "fxyz"
  Step1/1 -> Sum/2
  Step/1 -> Sum/1

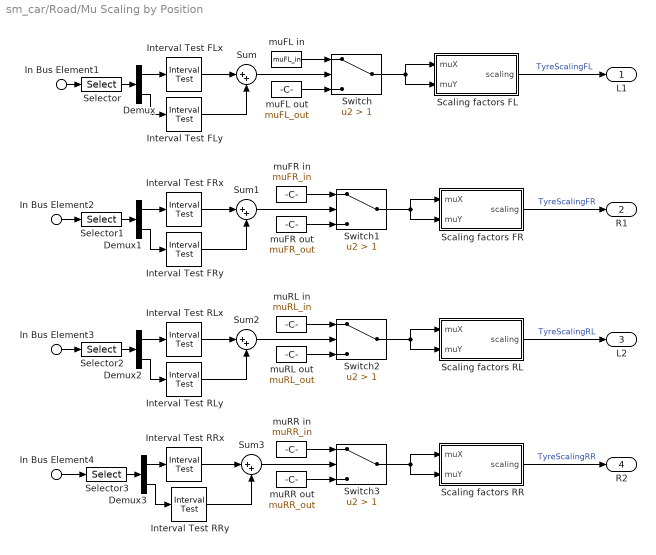
== system sm_car/Road/Mu Scaling by Position ==
  In Bus Element1 : Inport  PortName=Chassis  Element=WhlL1.xyz
  In Bus Element2 : Inport  PortName=Chassis  Element=WhlR1.xyz
  In Bus Element3 : Inport  PortName=Chassis  Element=WhlL2.xyz
  In Bus Element4 : Inport  PortName=Chassis  Element=WhlR2.xyz
  Demux{,1..3} (4 alike) : Demux  Outputs=2
  Interval Test FLx : simulink/Logic and Bit Operations/Interval Test  IntervalClosedRight=on  uplimit=intvX_FL_end  IntervalClosedLeft=on  lowlimit=intvX_FL_start  OutDataTypeStr=uint8
  Interval Test FLy : simulink/Logic and Bit Operations/Interval Test  IntervalClosedRight=on  uplimit=intvY_FL_end  IntervalClosedLeft=on  lowlimit=intvY_FL_start  OutDataTypeStr=uint8
  Interval Test FRx : simulink/Logic and Bit Operations/Interval Test  IntervalClosedRight=on  uplimit=intvX_FR_end  IntervalClosedLeft=on  lowlimit=intvX_FR_start  OutDataTypeStr=uint8
  Interval Test FRy : simulink/Logic and Bit Operations/Interval Test  IntervalClosedRight=on  uplimit=intvY_FR_end  IntervalClosedLeft=on  lowlimit=intvY_FR_start  OutDataTypeStr=uint8
  Interval Test RLx : simulink/Logic and Bit Operations/Interval Test  IntervalClosedRight=on  uplimit=intvX_RL_end  IntervalClosedLeft=on  lowlimit=intvX_RL_start  OutDataTypeStr=uint8
  Interval Test RLy : simulink/Logic and Bit Operations/Interval Test  IntervalClosedRight=on  uplimit=intvY_RL_end  IntervalClosedLeft=on  lowlimit=intvY_RL_start  OutDataTypeStr=uint8
  Interval Test RRx : simulink/Logic and Bit Operations/Interval Test  IntervalClosedRight=on  uplimit=intvX_RR_end  IntervalClosedLeft=on  lowlimit=intvX_RR_start  OutDataTypeStr=uint8
  Interval Test RRy : simulink/Logic and Bit Operations/Interval Test  IntervalClosedRight=on  uplimit=intvY_RR_end  IntervalClosedLeft=on  lowlimit=intvY_RR_start  OutDataTypeStr=uint8
  Scaling factors FL : Subsystem  mask{LKX=1, LKY=1, LKYC=1, LTR=1, LKZC=1}
      mask prompts: LKX "longitudinal slip stiffness"; LKY "cornering stiffness"; LKYC "camber stiffness"; LTR "pneumatic trail"; LKZC "camber torque stiffness"
  Scaling factors FR : Subsystem  mask{LKX=1, LKY=1, LKYC=1, LTR=1, LKZC=1}
      mask prompts: LKX "longitudinal slip stiffness"; LKY "cornering stiffness"; LKYC "camber stiffness"; LTR "pneumatic trail"; LKZC "camber torque stiffness"
  Scaling factors RL : Subsystem  mask{LKX=1, LKY=1, LKYC=1, LTR=1, LKZC=1}
      mask prompts: LKX "longitudinal slip stiffness"; LKY "cornering stiffness"; LKYC "camber stiffness"; LTR "pneumatic trail"; LKZC "camber torque stiffness"
  Scaling factors RR : Subsystem  mask{LKX=1, LKY=1, LKYC=1, LTR=1, LKZC=1}
      mask prompts: LKX "longitudinal slip stiffness"; LKY "cornering stiffness"; LKYC "camber stiffness"; LTR "pneumatic trail"; LKZC "camber torque stiffness"
  Selector{,1..3} (4 alike) : Selector  InputPortWidth=3  IndexOptions=Index vector (dialog)  Indices=[1 2]  OutputSizes=1
  Sum{,1..3} (4 alike) : Sum  Inputs=|++
  Switch : Switch  Criteria=u2 > Threshold  Threshold=1  ZeroCross=off  SaturateOnIntegerOverflow=off  InputSameDT=off
  Switch1 : Switch  Criteria=u2 > Threshold  Threshold=1  SaturateOnIntegerOverflow=off  InputSameDT=off
  Switch2 : Switch  Criteria=u2 > Threshold  Threshold=1  SaturateOnIntegerOverflow=off  InputSameDT=off
  Switch3 : Switch  Criteria=u2 > Threshold  Threshold=1  SaturateOnIntegerOverflow=off  InputSameDT=off
  muFL in : Constant  Value=muFL_in
  muFL out : Constant  Value=muFL_out
  muFR in : Constant  Value=muFR_in
  muFR out : Constant  Value=muFR_out
  muRL in : Constant  Value=muRL_in
  muRL out : Constant  Value=muRL_out
  muRR in : Constant  Value=muRR_in
  muRR out : Constant  Value=muRR_out
  L1 : Outport  VectorParamsAs1DForOutWhenUnconnected=off
  R1 : Outport  Port=2  VectorParamsAs1DForOutWhenUnconnected=off
  L2 : Outport  Port=3  VectorParamsAs1DForOutWhenUnconnected=off
  R2 : Outport  Port=4  VectorParamsAs1DForOutWhenUnconnected=off
  wires:
  Demux/1 -> Interval Test FLx/1
  Interval Test RRx/1 -> Sum3/1
  Demux3/2 -> Interval Test RRy/1
  Demux3/1 -> Interval Test RRx/1
  Sum3/1 -> Switch3/2
  Selector3/1 -> Demux3/1
  In Bus Element4/1 -> Selector3/1
  Interval Test RRy/1 -> Sum3/2
  Demux2/2 -> Interval Test RLy/1
  Selector2/1 -> Demux2/1
  Demux2/1 -> Interval Test RLx/1
  Interval Test RLy/1 -> Sum2/2
  Sum2/1 -> Switch2/2
  In Bus Element3/1 -> Selector2/1
  Interval Test RLx/1 -> Sum2/1
  Interval Test FRy/1 -> Sum1/2
  Selector1/1 -> Demux1/1
  Demux1/2 -> Interval Test FRy/1
  Sum1/1 -> Switch1/2
  Demux1/1 -> Interval Test FRx/1
  Interval Test FRx/1 -> Sum1/1
  Interval Test FLx/1 -> Sum/1
  Interval Test FLy/1 -> Sum/2
  Sum/1 -> Switch/2
  Demux/2 -> Interval Test FLy/1
  Selector/1 -> Demux/1
  muRR out/1 -> Switch3/3
  muRR in/1 -> Switch3/1
  Switch3/1 -> Scaling factors RR/2(muY), Scaling factors RR/1(muX)
  Scaling factors RR/1(scaling) -> R2/1  "TyreScalingRR"
  Scaling factors RL/1(scaling) -> L2/1  "TyreScalingRL"
  Switch2/1 -> Scaling factors RL/1(muX), Scaling factors RL/2(muY)
  muRL in/1 -> Switch2/1
  muRL out/1 -> Switch2/3
  muFR out/1 -> Switch1/3
  In Bus Element2/1 -> Selector1/1
  muFR in/1 -> Switch1/1
  Switch1/1 -> Scaling factors FR/2(muY), Scaling factors FR/1(muX)
  Scaling factors FR/1(scaling) -> R1/1  "TyreScalingFR"
  Scaling factors FL/1(scaling) -> L1/1  "TyreScalingFL"
  Switch/1 -> Scaling factors FL/1(muX), Scaling factors FL/2(muY)
  muFL out/1 -> Switch/3
  muFL in/1 -> Switch/1
  In Bus Element1/1 -> Selector/1

== system sm_car/Road/Road Surface Height ==
  Chassis : Inport
  None : Subsystem  VariantControl=None
  gz : Outport  VectorParamsAs1DForOutWhenUnconnected=off
  uvec : Outport  Port=2  VectorParamsAs1DForOutWhenUnconnected=off
